simulink model "kuka_sim"  (R2018b)
settings: Solver=VariableStepAuto  StartTime=0.0  StopTime=20  RelTol=1e-3
model workspace (MAT data in the model file):
  MCOS : class17 (value not decoded)
  MCOS : class17 (value not decoded)
  MCOS : class17 (value not decoded)
  MCOS : class17 (value not decoded)
  MCOS : class17 (value not decoded)
  MCOS : class17 (value not decoded)
  MCOS : class17 (value not decoded)
  I_C_1 = [0.00455  0  0; 0  0.00454  1e-05; 0  -1e-05  0.00029]
  I_C_2 = [0.00032  0  0; 0  0.0001  0; 0  0  0.00042]
  I_C_3 = [0.00223  -5e-05  7e-05; 5e-05  0.00219  7e-05; -7e-05  -7e-05  0.00073]
  I_C_4 = [0.03844  0.00088  -0.00112; -0.00088  0.01144  -0.00111; 0.00112  0.00111  0.04988]
  I_C_5 = [0.00277  -1e-05  1e-05; 1e-05  0.00284  0; -1e-05  0  0.00012]
  I_C_6 = [0.0005  -5e-05  -3e-05; 5e-05  0.00281  -4e-05; 3e-05  4e-05  0.00232]
  I_C_7 = [0.00795  0.00022  -0.00029; -0.00022  0.01089  -0.00029; 0.00029  0.00029  0.00294]
  MCOS : class17 (value not decoded)
  MCOS : class17 (value not decoded)
  MCOS : class17 (value not decoded)
  MCOS : class17 (value not decoded)
  MCOS : class17 (value not decoded)
  MCOS : class17 (value not decoded)
  MCOS : class17 (value not decoded)
  Pc_1 = [-0.00351; 0.0016; -0.03139]
  Pc_2 = [-0.00767; 0.16669; -0.00355]
  Pc_3 = [-0.00225; -0.03492; -0.02652]
  Pc_4 = [0.0002; -0.05268; 0.03818]
  Pc_5 = [5e-05; -0.00237; -0.21134]
  Pc_6 = [0.00049; 0.02019; -0.0275]
  Pc_7 = [-0.03466; -0.02324; 0.07138]
  MCOS : class17 (value not decoded)
  MCOS : class17 (value not decoded)
  MCOS : class17 (value not decoded)
  MCOS : class17 (value not decoded)
  MCOS : class17 (value not decoded)
  MCOS : class17 (value not decoded)
  MCOS : class17 (value not decoded)
  MCOS : class17 (value not decoded)
  MCOS : class17 (value not decoded)
  MCOS : class17 (value not decoded)
  MCOS : class17 (value not decoded)
  MCOS : class17 (value not decoded)
  MCOS : class17 (value not decoded)
  MCOS : class17 (value not decoded)
  MCOS : class17 (value not decoded)
  T_8_7 = [1 0 0 0 0 1 0 0 0 0 1 0 ... (16 elements, 4x4)]
  V_0 = [0; 0; 0]
  MCOS : class17 (value not decoded)
  MCOS : class17 (value not decoded)
  MCOS : class17 (value not decoded)
  MCOS : class17 (value not decoded)
  MCOS : class17 (value not decoded)
  MCOS : class17 (value not decoded)
  MCOS : class17 (value not decoded)
  MCOS : class17 (value not decoded)
  MCOS : class17 (value not decoded)
  MCOS : class17 (value not decoded)
  MCOS : class17 (value not decoded)
  MCOS : class17 (value not decoded)
  MCOS : class17 (value not decoded)
  MCOS : class17 (value not decoded)
  MCOS : class17 (value not decoded)
  MCOS : class17 (value not decoded)
  MCOS : class17 (value not decoded)
  MCOS : class17 (value not decoded)
  MCOS : class17 (value not decoded)
  MCOS : class17 (value not decoded)
  MCOS : class17 (value not decoded)
  MCOS : class17 (value not decoded)
  Var1 = 0
  W_0 = [0; 0; 0]
  W_0_dot = [0; 0; 0]
  MCOS : class17 (value not decoded)
  MCOS : class17 (value not decoded)
  MCOS : class17 (value not decoded)
  MCOS : class17 (value not decoded)
  MCOS : class17 (value not decoded)
  MCOS : class17 (value not decoded)
  MCOS : class17 (value not decoded)
  MCOS : class17 (value not decoded)
  MCOS : class17 (value not decoded)
  MCOS : class17 (value not decoded)
  MCOS : class17 (value not decoded)
  MCOS : class17 (value not decoded)
  MCOS : class17 (value not decoded)
  MCOS : class17 (value not decoded)
  a_0 = 0
  a_1 = 0
  a_2 = 0
  a_3 = 0
  a_4 = 0
  a_5 = 0
  a_6 = 0
  a_7 = 0
  alpha_0 = 0
  alpha_1 = 90
  alpha_2 = -90
  alpha_3 = -90
  alpha_4 = 90
  alpha_5 = 90
  alpha_6 = -90
  alpha_7 = 0
  d_1 = 0
  d_2 = 0
  d_3 = 0.4
  d_4 = 0
  d_5 = 0.39
  d_6 = 0
  d_7 = 0
  d_8 = 0
  MCOS : class17 (value not decoded)
  MCOS : class17 (value not decoded)
  MCOS : class17 (value not decoded)
  MCOS : class17 (value not decoded)
  MCOS : class17 (value not decoded)
  MCOS : class17 (value not decoded)
  MCOS : class17 (value not decoded)
  f_end = [0; 0; 0]
  MCOS : class17 (value not decoded)
  m1 = 3.94781
  m2 = 4.50275
  m3 = 2.4552
  m4 = 2.61155
  m5 = 3.41
  m6 = 3.38795
  m7 = 0.35432
  MCOS : class17 (value not decoded)
  MCOS : class17 (value not decoded)
  MCOS : class17 (value not decoded)
  MCOS : class17 (value not decoded)
  MCOS : class17 (value not decoded)
  MCOS : class17 (value not decoded)
  MCOS : class17 (value not decoded)
  n_end = [0; 0; 0]
  pi = 180
  MCOS : class17 (value not decoded)
  MCOS : class17 (value not decoded)
  MCOS : class17 (value not decoded)
  MCOS : class17 (value not decoded)
  MCOS : class17 (value not decoded)
  MCOS : class17 (value not decoded)
  MCOS : class17 (value not decoded)
  MCOS : class17 (value not decoded)
  MCOS : class17 (value not decoded)
  MCOS : class17 (value not decoded)
  MCOS : class17 (value not decoded)
  MCOS : class17 (value not decoded)
  MCOS : class17 (value not decoded)
  MCOS : class17 (value not decoded)
  MCOS : class17 (value not decoded)
  MCOS : class17 (value not decoded)
  MCOS : class17 (value not decoded)
  MCOS : class17 (value not decoded)
  MCOS : class17 (value not decoded)
  MCOS : class17 (value not decoded)
  MCOS : class17 (value not decoded)
  MCOS : class17 (value not decoded)
  MCOS : class17 (value not decoded)
  MCOS : class17 (value not decoded)
  MCOS : class17 (value not decoded)
  MCOS : class17 (value not decoded)
  MCOS : class17 (value not decoded)
  MCOS : class17 (value not decoded)
  MCOS : class17 (value not decoded)
  MCOS : class17 (value not decoded)
  MCOS : class17 (value not decoded)
  MCOS : class17 (value not decoded)
  MCOS : class17 (value not decoded)
  MCOS : class17 (value not decoded)
  MCOS : class17 (value not decoded)
  theta_8 = 0
(part 2 of 2)

== matlab function kuka_sim/MATLAB Function2 ==
  data: q input; torque output; q_dot input; q_des input; q_des_dot input; q_des_ddot input
function torque = fcn(q,q_dot,q_des,q_des_dot,q_des_ddot)

q_1 = q(1);
q_2 = q(2);
q_3 = q(3);
q_4 = q(4);

q_1_dot = q_dot(1);
q_2_dot = q_dot(2);
q_3_dot = q_dot(3);
q_4_dot = q_dot(4);

% q_1_ddot = q_ddot(1);
% q_2_ddot = q_ddot(2);
% q_3_ddot = q_ddot(3);
% q_4_ddot = q_ddot(4);

m11=cos(q_2)*(0.00415795377963*cos(q_2) + 0.005756821258825*sin(q_2) + 0.001993178216*cos(q_3)*sin(q_2) - 0.03195052591232*sin(q_2)*sin(q_3) + 1.0*cos(q_4)*(0.01524699328022*cos(q_2)*cos(q_4) - 0.000208924*cos(q_3)*sin(q_2) - 0.0008524847092*cos(q_2)*sin(q_4) + 0.00414266901372*sin(q_2)*sin(q_3) + 0.0008524847092*cos(q_3)*cos(q_4)*sin(q_2) + 0.01524699328022*cos(q_3)*sin(q_2)*sin(q_4) + 0.0398835916*cos(q_4)*sin(q_2)*sin(q_3)) + sin(q_4)*(0.0009075152908*cos(q_2)*cos(q_4) - 0.0550305816*cos(q_3)*sin(q_2) + 0.04949441641494*cos(q_2)*sin(q_4) - 0.0011399417958*sin(q_2)*sin(q_3) + 0.0398835916*sin(q_2)*sin(q_3)*sin(q_4) - 0.04949441641494*cos(q_3)*cos(q_4)*sin(q_2) + 0.0009075152908*cos(q_3)*sin(q_2)*sin(q_4))) + 1.0*sin(q_2)*(0.005756821258825*cos(q_2) + 0.12548815863615*sin(q_2) - 1.0*cos(q_3)*(0.000076501784*cos(q_2) + 0.01909410731264*cos(q_3)*sin(q_2) - 0.000242905064*sin(q_2)*sin(q_3) + 1.0*cos(q_4)*(0.0009075152908*cos(q_2)*cos(q_4) - 0.0550305816*cos(q_3)*sin(q_2) + 0.04949441641494*cos(q_2)*sin(q_4) - 0.0011399417958*sin(q_2)*sin(q_3) + 0.0398835916*sin(q_2)*sin(q_3)*sin(q_4) - 0.04949441641494*cos(q_3)*cos(q_4)*sin(q_2) + 0.0009075152908*cos(q_3)*sin(q_2)*sin(q_4)) - 1.0*sin(q_4)*(0.01524699328022*cos(q_2)*cos(q_4) - 0.000208924*cos(q_3)*sin(q_2) - 0.0008524847092*cos(q_2)*sin(q_4) + 0.00414266901372*sin(q_2)*sin(q_3) + 0.0008524847092*cos(q_3)*cos(q_4)*sin(q_2) + 0.01524699328022*cos(q_3)*sin(q_2)*sin(q_4) + 0.0398835916*cos(q_4)*sin(q_2)*sin(q_3))) + 1.0*sin(q_3)*(0.00220370768768*cos(q_2) + 0.00636266901372*cos(q_2)*cos(q_4) + 0.000142905064*cos(q_3)*sin(q_2) + 0.0011000582042*cos(q_2)*sin(q_4) + 0.0350120676028*sin(q_2)*sin(q_3) - 0.000208924*sin(q_2)*sin(q_3)*sin(q_4) - 0.0011000582042*cos(q_3)*cos(q_4)*sin(q_2) + 0.00636266901372*cos(q_3)*sin(q_2)*sin(q_4) + 0.0550305816*cos(q_4)*sin(q_2)*sin(q_3)) + 0.4*sin(q_3)*(cos(q_4)*(0.099708979*cos(q_2)*cos(q_4) + 0.137576454*sin(q_2)*sin(q_3) + 0.099708979*cos(q_3)*sin(q_2)*sin(q_4) + 1.04462*cos(q_4)*sin(q_2)*sin(q_3)) - 0.085735584*cos(q_2) + 0.916968096*sin(q_2)*sin(q_3) + 1.0*sin(q_4)*(0.099708979*cos(q_2)*sin(q_4) - 0.00052231*sin(q_2)*sin(q_3) + 1.04462*sin(q_2)*sin(q_3)*sin(q_4) - 0.099708979*cos(q_3)*cos(q_4)*sin(q_2))) + 0.4*cos(q_3)*(0.0055242*cos(q_2) - 0.00052231*cos(q_2)*cos(q_4) + 1.961588096*cos(q_3)*sin(q_2) - 0.137576454*cos(q_2)*sin(q_4) + 0.137576454*cos(q_3)*cos(q_4)*sin(q_2) - 0.00052231*cos(q_3)*sin(q_2)*sin(q_4))) + 0.00034874380758100000061534551321074;
m12=1.0*sin(q_2)*(1.0*cos(q_3)*(0.000242905064*cos(q_3) + 0.01909410731264*sin(q_3) - 1.0*cos(q_4)*(0.0550305816*sin(q_3) - 0.0011399417958*cos(q_3) + 0.0398835916*cos(q_3)*sin(q_4) + 0.04949441641494*cos(q_4)*sin(q_3) - 0.0009075152908*sin(q_3)*sin(q_4)) + 1.0*sin(q_4)*(0.00414266901372*cos(q_3) + 0.000208924*sin(q_3) + 0.0398835916*cos(q_3)*cos(q_4) - 0.0008524847092*cos(q_4)*sin(q_3) - 0.01524699328022*sin(q_3)*sin(q_4))) - 0.4*cos(q_3)*(1.961588096*sin(q_3) + 0.137576454*cos(q_4)*sin(q_3) - 0.00052231*sin(q_3)*sin(q_4)) + 0.4*sin(q_3)*(0.916968096*cos(q_3) + cos(q_4)*(0.137576454*cos(q_3) + 1.04462*cos(q_3)*cos(q_4) - 0.099708979*sin(q_3)*sin(q_4)) + 1.0*sin(q_4)*(1.04462*cos(q_3)*sin(q_4) - 0.00052231*cos(q_3) + 0.099708979*cos(q_4)*sin(q_3))) + 1.0*sin(q_3)*(0.0350120676028*cos(q_3) - 0.000142905064*sin(q_3) + 0.0550305816*cos(q_3)*cos(q_4) - 0.000208924*cos(q_3)*sin(q_4) + 0.0011000582042*cos(q_4)*sin(q_3) - 0.00636266901372*sin(q_3)*sin(q_4)) - 0.000122603128375) + cos(q_2)*(1.0*cos(q_4)*(0.00414266901372*cos(q_3) + 0.000208924*sin(q_3) + 0.0398835916*cos(q_3)*cos(q_4) - 0.0008524847092*cos(q_4)*sin(q_3) - 0.01524699328022*sin(q_3)*sin(q_4)) - 0.001993178216*sin(q_3) - 0.03195052591232*cos(q_3) + sin(q_4)*(0.0550305816*sin(q_3) - 0.0011399417958*cos(q_3) + 0.0398835916*cos(q_3)*sin(q_4) + 0.04949441641494*cos(q_4)*sin(q_3) - 0.0009075152908*sin(q_3)*sin(q_4)) + 0.002664500061125);
m13=cos(q_2)*(sin(q_4)*(0.0009075152908*cos(q_4) + 0.04949441641494*sin(q_4)) + 1.0*cos(q_4)*(0.01524699328022*cos(q_4) - 0.0008524847092*sin(q_4)) + 0.00373631604328) + 1.0*sin(q_2)*(1.0*sin(q_3)*(0.00636266901372*cos(q_4) + 0.0011000582042*sin(q_4) + 0.00220370768768) - 1.0*cos(q_3)*(1.0*cos(q_4)*(0.0009075152908*cos(q_4) + 0.04949441641494*sin(q_4)) - 1.0*sin(q_4)*(0.01524699328022*cos(q_4) - 0.0008524847092*sin(q_4)) + 0.000076501784) - 0.4*cos(q_3)*(0.00052231*cos(q_4) + 0.137576454*sin(q_4) - 0.0055242) + 0.4*sin(q_3)*(0.099708979*cos(q_4)^2 + 0.099708979*sin(q_4)^2 - 0.085735584));
m14=- 1.0*sin(q_2)*(0.05712763205872*sin(q_3) + 1.0*cos(q_3)*(0.0011399417958*cos(q_4) + 0.00414266901372*sin(q_4)) + 0.4*sin(q_3)*(0.137576454*cos(q_4) - 0.00052231*sin(q_4))) - cos(q_2)*(0.00414266901372*cos(q_4) - 0.0011399417958*sin(q_4));
m21=0.002664500061125*cos(q_2) - 0.000122603128375*sin(q_2) + sin(q_3)*(0.000076501784*cos(q_2) + 0.01909410731264*cos(q_3)*sin(q_2) - 0.000242905064*sin(q_2)*sin(q_3) + 1.0*cos(q_4)*(0.0009075152908*cos(q_2)*cos(q_4) - 0.0550305816*cos(q_3)*sin(q_2) + 0.04949441641494*cos(q_2)*sin(q_4) - 0.0011399417958*sin(q_2)*sin(q_3) + 0.0398835916*sin(q_2)*sin(q_3)*sin(q_4) - 0.04949441641494*cos(q_3)*cos(q_4)*sin(q_2) + 0.0009075152908*cos(q_3)*sin(q_2)*sin(q_4)) - 1.0*sin(q_4)*(0.01524699328022*cos(q_2)*cos(q_4) - 0.000208924*cos(q_3)*sin(q_2) - 0.0008524847092*cos(q_2)*sin(q_4) + 0.00414266901372*sin(q_2)*sin(q_3) + 0.0008524847092*cos(q_3)*cos(q_4)*sin(q_2) + 0.01524699328022*cos(q_3)*sin(q_2)*sin(q_4) + 0.0398835916*cos(q_4)*sin(q_2)*sin(q_3))) + 1.0*cos(q_3)*(0.00220370768768*cos(q_2) + 0.00636266901372*cos(q_2)*cos(q_4) + 0.000142905064*cos(q_3)*sin(q_2) + 0.0011000582042*cos(q_2)*sin(q_4) + 0.0350120676028*sin(q_2)*sin(q_3) - 0.000208924*sin(q_2)*sin(q_3)*sin(q_4) - 0.0011000582042*cos(q_3)*cos(q_4)*sin(q_2) + 0.00636266901372*cos(q_3)*sin(q_2)*sin(q_4) + 0.0550305816*cos(q_4)*sin(q_2)*sin(q_3)) + 0.4*cos(q_3)*(cos(q_4)*(0.099708979*cos(q_2)*cos(q_4) + 0.137576454*sin(q_2)*sin(q_3) + 0.099708979*cos(q_3)*sin(q_2)*sin(q_4) + 1.04462*cos(q_4)*sin(q_2)*sin(q_3)) - 0.085735584*cos(q_2) + 0.916968096*sin(q_2)*sin(q_3) + 1.0*sin(q_4)*(0.099708979*cos(q_2)*sin(q_4) - 0.00052231*sin(q_2)*sin(q_3) + 1.04462*sin(q_2)*sin(q_3)*sin(q_4) - 0.099708979*cos(q_3)*cos(q_4)*sin(q_2))) - 0.4*sin(q_3)*(0.0055242*cos(q_2) - 0.00052231*cos(q_2)*cos(q_4) + 1.961588096*cos(q_3)*sin(q_2) - 0.137576454*cos(q_2)*sin(q_4) + 0.137576454*cos(q_3)*cos(q_4)*sin(q_2) - 0.00052231*cos(q_3)*sin(q_2)*sin(q_4));
m22=0.4*sin(q_3)*(1.961588096*sin(q_3) + 0.137576454*cos(q_4)*sin(q_3) - 0.00052231*sin(q_3)*sin(q_4)) - sin(q_3)*(0.000242905064*cos(q_3) + 0.01909410731264*sin(q_3) - 1.0*cos(q_4)*(0.0550305816*sin(q_3) - 0.0011399417958*cos(q_3) + 0.0398835916*cos(q_3)*sin(q_4) + 0.04949441641494*cos(q_4)*sin(q_3) - 0.0009075152908*sin(q_3)*sin(q_4)) + 1.0*sin(q_4)*(0.00414266901372*cos(q_3) + 0.000208924*sin(q_3) + 0.0398835916*cos(q_3)*cos(q_4) - 0.0008524847092*cos(q_4)*sin(q_3) - 0.01524699328022*sin(q_3)*sin(q_4))) + 0.4*cos(q_3)*(0.916968096*cos(q_3) + cos(q_4)*(0.137576454*cos(q_3) + 1.04462*cos(q_3)*cos(q_4) - 0.099708979*sin(q_3)*sin(q_4)) + 1.0*sin(q_4)*(1.04462*cos(q_3)*sin(q_4) - 0.00052231*cos(q_3) + 0.099708979*cos(q_4)*sin(q_3))) + 1.0*cos(q_3)*(0.0350120676028*cos(q_3) - 0.000142905064*sin(q_3) + 0.0550305816*cos(q_3)*cos(q_4) - 0.000208924*cos(q_3)*sin(q_4) + 0.0011000582042*cos(q_4)*sin(q_3) - 0.00636266901372*sin(q_3)*sin(q_4)) + 0.12579630455875;
m23=0.4*sin(q_3)*(0.00052231*cos(q_4) + 0.137576454*sin(q_4) - 0.0055242) + 1.0*cos(q_3)*(0.00636266901372*cos(q_4) + 0.0011000582042*sin(q_4) + 0.00220370768768) + sin(q_3)*(1.0*cos(q_4)*(0.0009075152908*cos(q_4) + 0.04949441641494*sin(q_4)) - 1.0*sin(q_4)*(0.01524699328022*cos(q_4) - 0.0008524847092*sin(q_4)) + 0.000076501784) + 0.4*cos(q_3)*(0.099708979*cos(q_4)^2 + 0.099708979*sin(q_4)^2 - 0.085735584);
m24=sin(q_3)*(0.0011399417958*cos(q_4) + 0.00414266901372*sin(q_4)) - 0.4*cos(q_3)*(0.137576454*cos(q_4) - 0.00052231*sin(q_4)) - 0.05712763205872*cos(q_3);
m31=0.00373631604328*cos(q_2) + 0.001993178216*cos(q_3)*sin(q_2) - 0.03195052591232*sin(q_2)*sin(q_3) + 1.0*cos(q_4)*(0.01524699328022*cos(q_2)*cos(q_4) - 0.000208924*cos(q_3)*sin(q_2) - 0.0008524847092*cos(q_2)*sin(q_4) + 0.00414266901372*sin(q_2)*sin(q_3) + 0.0008524847092*cos(q_3)*cos(q_4)*sin(q_2) + 0.01524699328022*cos(q_3)*sin(q_2)*sin(q_4) + 0.0398835916*cos(q_4)*sin(q_2)*sin(q_3)) + sin(q_4)*(0.0009075152908*cos(q_2)*cos(q_4) - 0.0550305816*cos(q_3)*sin(q_2) + 0.04949441641494*cos(q_2)*sin(q_4) - 0.0011399417958*sin(q_2)*sin(q_3) + 0.0398835916*sin(q_2)*sin(q_3)*sin(q_4) - 0.04949441641494*cos(q_3)*cos(q_4)*sin(q_2) + 0.0009075152908*cos(q_3)*sin(q_2)*sin(q_4));
m32=1.0*cos(q_4)*(0.00414266901372*cos(q_3) + 0.000208924*sin(q_3) + 0.0398835916*cos(q_3)*cos(q_4) - 0.0008524847092*cos(q_4)*sin(q_3) - 0.01524699328022*sin(q_3)*sin(q_4)) - 0.001993178216*sin(q_3) - 0.03195052591232*cos(q_3) + sin(q_4)*(0.0550305816*sin(q_3) - 0.0011399417958*cos(q_3) + 0.0398835916*cos(q_3)*sin(q_4) + 0.04949441641494*cos(q_4)*sin(q_3) - 0.0009075152908*sin(q_3)*sin(q_4));
m33=sin(q_4)*(0.0009075152908*cos(q_4) + 0.04949441641494*sin(q_4)) + 1.0*cos(q_4)*(0.01524699328022*cos(q_4) - 0.0008524847092*sin(q_4)) + 0.00373631604328;
m34=0.0011399417958*sin(q_4) - 0.00414266901372*cos(q_4);
m41=0.000208924*sin(q_2)*sin(q_3)*sin(q_4) - 0.0011000582042*cos(q_2)*sin(q_4) - 0.05712763205872*sin(q_2)*sin(q_3) - 0.00636266901372*cos(q_2)*cos(q_4) + 0.0011000582042*cos(q_3)*cos(q_4)*sin(q_2) - 0.00636266901372*cos(q_3)*sin(q_2)*sin(q_4) - 0.0550305816*cos(q_4)*sin(q_2)*sin(q_3);
m42=0.000208924*cos(q_3)*sin(q_4) - 0.0550305816*cos(q_3)*cos(q_4) - 0.05712763205872*cos(q_3) - 0.0011000582042*cos(q_4)*sin(q_3) + 0.00636266901372*sin(q_3)*sin(q_4);
m43=- 0.00636266901372*cos(q_4) - 0.0011000582042*sin(q_4);
m44=0.05712763205872;

M=[m11 m12 m13 m14;m21 m22 m23 m24;m31 m32 m33 m34;m41 m42 m43 m44];

c11=0;
c12=- cos(q_2)*(0.005756821258825*q_1*sin(q_2)^2 + 0.0055242*cos(q_3)*(0.4*q_1*sin(q_2)^2 - 0.4*q_2*cos(q_2)) - 0.085735584*sin(q_3)*(0.4*q_1*sin(q_2)^2 - 0.4*q_2*cos(q_2)) + 1.0*cos(q_4)*(0.01524699328022*cos(q_4)*(1.0*q_2*sin(q_2) + 1.0*q_1*cos(q_2)*sin(q_2)) - 0.00052231*cos(q_3)*(0.4*q_1*sin(q_2)^2 - 0.4*q_2*cos(q_2)) - 0.0008524847092*sin(q_4)*(1.0*q_2*sin(q_2) + 1.0*q_1*cos(q_2)*sin(q_2)) + 0.00414266901372*sin(q_3)*(1.0*q_1*sin(q_2)^2 - 1.0*q_2*cos(q_2)) + 0.0008524847092*cos(q_3)*cos(q_4)*(1.0*q_1*sin(q_2)^2 - 1.0*q_2*cos(q_2)) + 0.01524699328022*cos(q_3)*sin(q_4)*(1.0*q_1*sin(q_2)^2 - 1.0*q_2*cos(q_2)) + 0.099708979*cos(q_4)*sin(q_3)*(0.4*q_1*sin(q_2)^2 - 0.4*q_2*cos(q_2))) + sin(q_4)*(0.0009075152908*cos(q_4)*(1.0*q_2*sin(q_2) + 1.0*q_1*cos(q_2)*sin(q_2)) - 0.137576454*cos(q_3)*(0.4*q_1*sin(q_2)^2 - 0.4*q_2*cos(q_2)) + 0.04949441641494*sin(q_4)*(1.0*q_2*sin(q_2) + 1.0*q_1*cos(q_2)*sin(q_2)) - 0.0011399417958*sin(q_3)*(1.0*q_1*sin(q_2)^2 - 1.0*q_2*cos(q_2)) + 0.099708979*sin(q_3)*sin(q_4)*(0.4*q_1*sin(q_2)^2 - 0.4*q_2*cos(q_2)) - 0.04949441641494*cos(q_3)*cos(q_4)*(1.0*q_1*sin(q_2)^2 - 1.0*q_2*cos(q_2)) + 0.0009075152908*cos(q_3)*sin(q_4)*(1.0*q_1*sin(q_2)^2 - 1.0*q_2*cos(q_2))) - 0.005756821258825*q_2*cos(q_2) + 0.00415795377963*q_2*sin(q_2) - 0.000216501784*cos(q_3)*(1.0*q_1*sin(q_2)^2 - 1.0*q_2*cos(q_2)) + 0.00234370768768*sin(q_3)*(1.0*q_1*sin(q_2)^2 - 1.0*q_2*cos(q_2)) + 0.00415795377963*q_1*cos(q_2)*sin(q_2)) - 1.0*sin(q_2)*(0.12548815863615*q_1*sin(q_2)^2 + 0.4*cos(q_3)*(5.06675*cos(q_3)*(0.4*q_1*sin(q_2)^2 - 0.4*q_2*cos(q_2)) - 0.00052231*cos(q_4)*(1.0*q_2*sin(q_2) + 1.0*q_1*cos(q_2)*sin(q_2)) - 0.137576454*sin(q_4)*(1.0*q_2*sin(q_2) + 1.0*q_1*cos(q_2)*sin(q_2)) + 0.0055242*q_2*sin(q_2) - 0.065111904*cos(q_3)*(1.0*q_1*sin(q_2)^2 - 1.0*q_2*cos(q_2)) + 0.0055242*q_1*cos(q_2)*sin(q_2) + 0.137576454*cos(q_3)*cos(q_4)*(1.0*q_1*sin(q_2)^2 - 1.0*q_2*cos(q_2)) - 0.00052231*cos(q_3)*sin(q_4)*(1.0*q_1*sin(q_2)^2 - 1.0*q_2*cos(q_2))) + 0.4*sin(q_3)*(2.4552*sin(q_3)*(0.4*q_1*sin(q_2)^2 - 0.4*q_2*cos(q_2)) - 0.085735584*q_2*sin(q_2) - 0.065111904*sin(q_3)*(1.0*q_1*sin(q_2)^2 - 1.0*q_2*cos(q_2)) + cos(q_4)*(0.099708979*cos(q_4)*(1.0*q_2*sin(q_2) + 1.0*q_1*cos(q_2)*sin(q_2)) + 0.137576454*sin(q_3)*(1.0*q_1*sin(q_2)^2 - 1.0*q_2*cos(q_2)) + 0.099708979*cos(q_3)*sin(q_4)*(1.0*q_1*sin(q_2)^2 - 1.0*q_2*cos(q_2)) + 2.61155*cos(q_4)*sin(q_3)*(0.4*q_1*sin(q_2)^2 - 0.4*q_2*cos(q_2))) + 1.0*sin(q_4)*(0.099708979*sin(q_4)*(1.0*q_2*sin(q_2) + 1.0*q_1*cos(q_2)*sin(q_2)) - 0.00052231*sin(q_3)*(1.0*q_1*sin(q_2)^2 - 1.0*q_2*cos(q_2)) + 2.61155*sin(q_3)*sin(q_4)*(0.4*q_1*sin(q_2)^2 - 0.4*q_2*cos(q_2)) - 0.099708979*cos(q_3)*cos(q_4)*(1.0*q_1*sin(q_2)^2 - 1.0*q_2*cos(q_2))) - 0.085735584*q_1*cos(q_2)*sin(q_2)) + 1.0*sin(q_3)*(0.00636266901372*cos(q_4)*(1.0*q_2*sin(q_2) + 1.0*q_1*cos(q_2)*sin(q_2)) - 0.065111904*sin(q_3)*(0.4*q_1*sin(q_2)^2 - 0.4*q_2*cos(q_2)) + 0.0011000582042*sin(q_4)*(1.0*q_2*sin(q_2) + 1.0*q_1*cos(q_2)*sin(q_2)) + 0.00220370768768*q_2*sin(q_2) + 0.000142905064*cos(q_3)*(1.0*q_1*sin(q_2)^2 - 1.0*q_2*cos(q_2)) + 0.0610568292028*sin(q_3)*(1.0*q_1*sin(q_2)^2 - 1.0*q_2*cos(q_2)) - 0.00052231*sin(q_3)*sin(q_4)*(0.4*q_1*sin(q_2)^2 - 0.4*q_2*cos(q_2)) + 0.00220370768768*q_1*cos(q_2)*sin(q_2) - 0.0011000582042*cos(q_3)*cos(q_4)*(1.0*q_1*sin(q_2)^2 - 1.0*q_2*cos(q_2)) + 0.00636266901372*cos(q_3)*sin(q_4)*(1.0*q_1*sin(q_2)^2 - 1.0*q_2*cos(q_2)) + 0.137576454*cos(q_4)*sin(q_3)*(0.4*q_1*sin(q_2)^2 - 0.4*q_2*cos(q_2))) - 0.12548815863615*q_2*cos(q_2) + 0.005756821258825*q_2*sin(q_2) - 1.0*cos(q_3)*(0.065111904*cos(q_3)*(0.4*q_1*sin(q_2)^2 - 0.4*q_2*cos(q_2)) + 1.0*cos(q_4)*(0.0009075152908*cos(q_4)*(1.0*q_2*sin(q_2) + 1.0*q_1*cos(q_2)*sin(q_2)) - 0.137576454*cos(q_3)*(0.4*q_1*sin(q_2)^2 - 0.4*q_2*cos(q_2)) + 0.04949441641494*sin(q_4)*(1.0*q_2*sin(q_2) + 1.0*q_1*cos(q_2)*sin(q_2)) - 0.0011399417958*sin(q_3)*(1.0*q_1*sin(q_2)^2 - 1.0*q_2*cos(q_2)) + 0.099708979*sin(q_3)*sin(q_4)*(0.4*q_1*sin(q_2)^2 - 0.4*q_2*cos(q_2)) - 0.04949441641494*cos(q_3)*cos(q_4)*(1.0*q_1*sin(q_2)^2 - 1.0*q_2*cos(q_2)) + 0.0009075152908*cos(q_3)*sin(q_4)*(1.0*q_1*sin(q_2)^2 - 1.0*q_2*cos(q_2))) - 1.0*sin(q_4)*(0.01524699328022*cos(q_4)*(1.0*q_2*sin(q_2) + 1.0*q_1*cos(q_2)*sin(q_2)) - 0.00052231*cos(q_3)*(0.4*q_1*sin(q_2)^2 - 0.4*q_2*cos(q_2)) - 0.0008524847092*sin(q_4)*(1.0*q_2*sin(q_2) + 1.0*q_1*cos(q_2)*sin(q_2)) + 0.00414266901372*sin(q_3)*(1.0*q_1*sin(q_2)^2 - 1.0*q_2*cos(q_2)) + 0.0008524847092*cos(q_3)*cos(q_4)*(1.0*q_1*sin(q_2)^2 - 1.0*q_2*cos(q_2)) + 0.01524699328022*cos(q_3)*sin(q_4)*(1.0*q_1*sin(q_2)^2 - 1.0*q_2*cos(q_2)) + 0.099708979*cos(q_4)*sin(q_3)*(0.4*q_1*sin(q_2)^2 - 0.4*q_2*cos(q_2))) + 0.000076501784*q_2*sin(q_2) - 0.00695065428736*cos(q_3)*(1.0*q_1*sin(q_2)^2 - 1.0*q_2*cos(q_2)) - 0.000242905064*sin(q_3)*(1.0*q_1*sin(q_2)^2 - 1.0*q_2*cos(q_2)) + 0.000076501784*q_1*cos(q_2)*sin(q_2)) + 0.005756821258825*q_1*cos(q_2)*sin(q_2));
c13=- 1.0*sin(q_2)*(0.4*cos(q_3)*(0.065111904*sin(q_3)*(q_2*sin(q_3) - 1.0*q_1*cos(q_3)*sin(q_2)) - 0.065111904*cos(q_3)*(q_3 + q_1*cos(q_2)) - 0.137576454*cos(q_4)*(1.0*sin(q_3)*(q_2*sin(q_3) - 1.0*q_1*cos(q_3)*sin(q_2)) - 1.0*cos(q_3)*(q_3 + q_1*cos(q_2))) + 0.00052231*sin(q_4)*(1.0*sin(q_3)*(q_2*sin(q_3) - 1.0*q_1*cos(q_3)*sin(q_2)) - 1.0*cos(q_3)*(q_3 + q_1*cos(q_2)))) + 1.0*sin(q_3)*(0.0610568292028*cos(q_3)*(q_2*sin(q_3) - 1.0*q_1*cos(q_3)*sin(q_2)) - 0.000142905064*sin(q_3)*(q_2*sin(q_3) - 1.0*q_1*cos(q_3)*sin(q_2)) + 0.000142905064*cos(q_3)*(q_3 + q_1*cos(q_2)) + 0.0610568292028*sin(q_3)*(q_3 + q_1*cos(q_2)) + 0.0011000582042*cos(q_4)*(1.0*sin(q_3)*(q_2*sin(q_3) - 1.0*q_1*cos(q_3)*sin(q_2)) - 1.0*cos(q_3)*(q_3 + q_1*cos(q_2))) - 0.00636266901372*sin(q_4)*(1.0*sin(q_3)*(q_2*sin(q_3) - 1.0*q_1*cos(q_3)*sin(q_2)) - 1.0*cos(q_3)*(q_3 + q_1*cos(q_2)))) - 0.4*sin(q_3)*(0.065111904*cos(q_3)*(q_2*sin(q_3) - 1.0*q_1*cos(q_3)*sin(q_2)) + 1.0*sin(q_4)*(0.00052231*cos(q_3)*(q_2*sin(q_3) - 1.0*q_1*cos(q_3)*sin(q_2)) + 0.00052231*sin(q_3)*(q_3 + q_1*cos(q_2)) - 0.099708979*cos(q_4)*(1.0*sin(q_3)*(q_2*sin(q_3) - 1.0*q_1*cos(q_3)*sin(q_2)) - 1.0*cos(q_3)*(q_3 + q_1*cos(q_2)))) - cos(q_4)*(0.137576454*cos(q_3)*(q_2*sin(q_3) - 1.0*q_1*cos(q_3)*sin(q_2)) + 0.137576454*sin(q_3)*(q_3 + q_1*cos(q_2)) - 0.099708979*sin(q_4)*(1.0*sin(q_3)*(q_2*sin(q_3) - 1.0*q_1*cos(q_3)*sin(q_2)) - 1.0*cos(q_3)*(q_3 + q_1*cos(q_2)))) + 0.065111904*sin(q_3)*(q_3 + q_1*cos(q_2))) + 1.0*cos(q_3)*(0.000242905064*cos(q_3)*(q_2*sin(q_3) - 1.0*q_1*cos(q_3)*sin(q_2)) - 0.00695065428736*sin(q_3)*(q_2*sin(q_3) - 1.0*q_1*cos(q_3)*sin(q_2)) + 1.0*cos(q_4)*(0.0011399417958*cos(q_3)*(q_2*sin(q_3) - 1.0*q_1*cos(q_3)*sin(q_2)) + 0.0011399417958*sin(q_3)*(q_3 + q_1*cos(q_2)) - 0.04949441641494*cos(q_4)*(1.0*sin(q_3)*(q_2*sin(q_3) - 1.0*q_1*cos(q_3)*sin(q_2)) - 1.0*cos(q_3)*(q_3 + q_1*cos(q_2))) + 0.0009075152908*sin(q_4)*(1.0*sin(q_3)*(q_2*sin(q_3) - 1.0*q_1*cos(q_3)*sin(q_2)) - 1.0*cos(q_3)*(q_3 + q_1*cos(q_2)))) + 0.00695065428736*cos(q_3)*(q_3 + q_1*cos(q_2)) + 1.0*sin(q_4)*(0.00414266901372*cos(q_3)*(q_2*sin(q_3) - 1.0*q_1*cos(q_3)*sin(q_2)) + 0.00414266901372*sin(q_3)*(q_3 + q_1*cos(q_2)) - 0.0008524847092*cos(q_4)*(1.0*sin(q_3)*(q_2*sin(q_3) - 1.0*q_1*cos(q_3)*sin(q_2)) - 1.0*cos(q_3)*(q_3 + q_1*cos(q_2))) - 0.01524699328022*sin(q_4)*(1.0*sin(q_3)*(q_2*sin(q_3) - 1.0*q_1*cos(q_3)*sin(q_2)) - 1.0*cos(q_3)*(q_3 + q_1*cos(q_2)))) + 0.000242905064*sin(q_3)*(q_3 + q_1*cos(q_2)))) - cos(q_2)*(0.00234370768768*cos(q_3)*(q_2*sin(q_3) - 1.0*q_1*cos(q_3)*sin(q_2)) + 0.000216501784*sin(q_3)*(q_2*sin(q_3) - 1.0*q_1*cos(q_3)*sin(q_2)) + 1.0*cos(q_4)*(0.00414266901372*cos(q_3)*(q_2*sin(q_3) - 1.0*q_1*cos(q_3)*sin(q_2)) + 0.00414266901372*sin(q_3)*(q_3 + q_1*cos(q_2)) - 0.0008524847092*cos(q_4)*(1.0*sin(q_3)*(q_2*sin(q_3) - 1.0*q_1*cos(q_3)*sin(q_2)) - 1.0*cos(q_3)*(q_3 + q_1*cos(q_2))) - 0.01524699328022*sin(q_4)*(1.0*sin(q_3)*(q_2*sin(q_3) - 1.0*q_1*cos(q_3)*sin(q_2)) - 1.0*cos(q_3)*(q_3 + q_1*cos(q_2)))) - 0.000216501784*cos(q_3)*(q_3 + q_1*cos(q_2)) - sin(q_4)*(0.0011399417958*cos(q_3)*(q_2*sin(q_3) - 1.0*q_1*cos(q_3)*sin(q_2)) + 0.0011399417958*sin(q_3)*(q_3 + q_1*cos(q_2)) - 0.04949441641494*cos(q_4)*(1.0*sin(q_3)*(q_2*sin(q_3) - 1.0*q_1*cos(q_3)*sin(q_2)) - 1.0*cos(q_3)*(q_3 + q_1*cos(q_2))) + 0.0009075152908*sin(q_4)*(1.0*sin(q_3)*(q_2*sin(q_3) - 1.0*q_1*cos(q_3)*sin(q_2)) - 1.0*cos(q_3)*(q_3 + q_1*cos(q_2)))) + 0.00234370768768*sin(q_3)*(q_3 + q_1*cos(q_2)));
c14=1.0*sin(q_2)*(1.0*cos(q_3)*(1.0*sin(q_4)*(0.0008524847092*sin(q_4)*(cos(q_4)*(q_2*sin(q_3) - 1.0*q_1*cos(q_3)*sin(q_2)) + sin(q_4)*(q_3 + q_1*cos(q_2))) - 0.01524699328022*cos(q_4)*(cos(q_4)*(q_2*sin(q_3) - 1.0*q_1*cos(q_3)*sin(q_2)) + sin(q_4)*(q_3 + q_1*cos(q_2))) + 0.0008524847092*cos(q_4)*(q_2*cos(q_3) - 1.0*q_4 + q_1*sin(q_2)*sin(q_3)) + 0.01524699328022*sin(q_4)*(q_2*cos(q_3) - 1.0*q_4 + q_1*sin(q_2)*sin(q_3))) + 1.0*cos(q_4)*(0.0009075152908*cos(q_4)*(cos(q_4)*(q_2*sin(q_3) - 1.0*q_1*cos(q_3)*sin(q_2)) + sin(q_4)*(q_3 + q_1*cos(q_2))) + 0.04949441641494*sin(q_4)*(cos(q_4)*(q_2*sin(q_3) - 1.0*q_1*cos(q_3)*sin(q_2)) + sin(q_4)*(q_3 + q_1*cos(q_2))) + 0.04949441641494*cos(q_4)*(q_2*cos(q_3) - 1.0*q_4 + q_1*sin(q_2)*sin(q_3)) - 0.0009075152908*sin(q_4)*(q_2*cos(q_3) - 1.0*q_4 + q_1*sin(q_2)*sin(q_3)))) + 0.4*cos(q_3)*(0.00052231*cos(q_4)*(cos(q_4)*(q_2*sin(q_3) - 1.0*q_1*cos(q_3)*sin(q_2)) + sin(q_4)*(q_3 + q_1*cos(q_2))) + 0.137576454*sin(q_4)*(cos(q_4)*(q_2*sin(q_3) - 1.0*q_1*cos(q_3)*sin(q_2)) + sin(q_4)*(q_3 + q_1*cos(q_2))) + 0.137576454*cos(q_4)*(q_2*cos(q_3) - 1.0*q_4 + q_1*sin(q_2)*sin(q_3)) - 0.00052231*sin(q_4)*(q_2*cos(q_3) - 1.0*q_4 + q_1*sin(q_2)*sin(q_3))) - 0.4*sin(q_3)*(cos(q_4)*(0.099708979*cos(q_4)*(cos(q_4)*(q_2*sin(q_3) - 1.0*q_1*cos(q_3)*sin(q_2)) + sin(q_4)*(q_3 + q_1*cos(q_2))) - 0.099708979*sin(q_4)*(q_2*cos(q_3) - 1.0*q_4 + q_1*sin(q_2)*sin(q_3))) + 1.0*sin(q_4)*(0.099708979*sin(q_4)*(cos(q_4)*(q_2*sin(q_3) - 1.0*q_1*cos(q_3)*sin(q_2)) + sin(q_4)*(q_3 + q_1*cos(q_2))) + 0.099708979*cos(q_4)*(q_2*cos(q_3) - 1.0*q_4 + q_1*sin(q_2)*sin(q_3)))) - 1.0*sin(q_3)*(0.00636266901372*cos(q_4)*(cos(q_4)*(q_2*sin(q_3) - 1.0*q_1*cos(q_3)*sin(q_2)) + sin(q_4)*(q_3 + q_1*cos(q_2))) + 0.0011000582042*sin(q_4)*(cos(q_4)*(q_2*sin(q_3) - 1.0*q_1*cos(q_3)*sin(q_2)) + sin(q_4)*(q_3 + q_1*cos(q_2))) + 0.0011000582042*cos(q_4)*(q_2*cos(q_3) - 1.0*q_4 + q_1*sin(q_2)*sin(q_3)) - 0.00636266901372*sin(q_4)*(q_2*cos(q_3) - 1.0*q_4 + q_1*sin(q_2)*sin(q_3)))) - cos(q_2)*(sin(q_4)*(0.0009075152908*cos(q_4)*(cos(q_4)*(q_2*sin(q_3) - 1.0*q_1*cos(q_3)*sin(q_2)) + sin(q_4)*(q_3 + q_1*cos(q_2))) + 0.04949441641494*sin(q_4)*(cos(q_4)*(q_2*sin(q_3) - 1.0*q_1*cos(q_3)*sin(q_2)) + sin(q_4)*(q_3 + q_1*cos(q_2))) + 0.04949441641494*cos(q_4)*(q_2*cos(q_3) - 1.0*q_4 + q_1*sin(q_2)*sin(q_3)) - 0.0009075152908*sin(q_4)*(q_2*cos(q_3) - 1.0*q_4 + q_1*sin(q_2)*sin(q_3))) - 1.0*cos(q_4)*(0.0008524847092*sin(q_4)*(cos(q_4)*(q_2*sin(q_3) - 1.0*q_1*cos(q_3)*sin(q_2)) + sin(q_4)*(q_3 + q_1*cos(q_2))) - 0.01524699328022*cos(q_4)*(cos(q_4)*(q_2*sin(q_3) - 1.0*q_1*cos(q_3)*sin(q_2)) + sin(q_4)*(q_3 + q_1*cos(q_2))) + 0.0008524847092*cos(q_4)*(q_2*cos(q_3) - 1.0*q_4 + q_1*sin(q_2)*sin(q_3)) + 0.01524699328022*sin(q_4)*(q_2*cos(q_3) - 1.0*q_4 + q_1*sin(q_2)*sin(q_3))));
c21=0;
c22=0.000122603128375*q_1*sin(q_2)^2 + 0.4*sin(q_3)*(5.06675*cos(q_3)*(0.4*q_1*sin(q_2)^2 - 0.4*q_2*cos(q_2)) - 0.00052231*cos(q_4)*(1.0*q_2*sin(q_2) + 1.0*q_1*cos(q_2)*sin(q_2)) - 0.137576454*sin(q_4)*(1.0*q_2*sin(q_2) + 1.0*q_1*cos(q_2)*sin(q_2)) + 0.0055242*q_2*sin(q_2) - 0.065111904*cos(q_3)*(1.0*q_1*sin(q_2)^2 - 1.0*q_2*cos(q_2)) + 0.0055242*q_1*cos(q_2)*sin(q_2) + 0.137576454*cos(q_3)*cos(q_4)*(1.0*q_1*sin(q_2)^2 - 1.0*q_2*cos(q_2)) - 0.00052231*cos(q_3)*sin(q_4)*(1.0*q_1*sin(q_2)^2 - 1.0*q_2*cos(q_2))) - 0.4*cos(q_3)*(2.4552*sin(q_3)*(0.4*q_1*sin(q_2)^2 - 0.4*q_2*cos(q_2)) - 0.085735584*q_2*sin(q_2) - 0.065111904*sin(q_3)*(1.0*q_1*sin(q_2)^2 - 1.0*q_2*cos(q_2)) + cos(q_4)*(0.099708979*cos(q_4)*(1.0*q_2*sin(q_2) + 1.0*q_1*cos(q_2)*sin(q_2)) + 0.137576454*sin(q_3)*(1.0*q_1*sin(q_2)^2 - 1.0*q_2*cos(q_2)) + 0.099708979*cos(q_3)*sin(q_4)*(1.0*q_1*sin(q_2)^2 - 1.0*q_2*cos(q_2)) + 2.61155*cos(q_4)*sin(q_3)*(0.4*q_1*sin(q_2)^2 - 0.4*q_2*cos(q_2))) + 1.0*sin(q_4)*(0.099708979*sin(q_4)*(1.0*q_2*sin(q_2) + 1.0*q_1*cos(q_2)*sin(q_2)) - 0.00052231*sin(q_3)*(1.0*q_1*sin(q_2)^2 - 1.0*q_2*cos(q_2)) + 2.61155*sin(q_3)*sin(q_4)*(0.4*q_1*sin(q_2)^2 - 0.4*q_2*cos(q_2)) - 0.099708979*cos(q_3)*cos(q_4)*(1.0*q_1*sin(q_2)^2 - 1.0*q_2*cos(q_2))) - 0.085735584*q_1*cos(q_2)*sin(q_2)) - 1.0*cos(q_3)*(0.00636266901372*cos(q_4)*(1.0*q_2*sin(q_2) + 1.0*q_1*cos(q_2)*sin(q_2)) - 0.065111904*sin(q_3)*(0.4*q_1*sin(q_2)^2 - 0.4*q_2*cos(q_2)) + 0.0011000582042*sin(q_4)*(1.0*q_2*sin(q_2) + 1.0*q_1*cos(q_2)*sin(q_2)) + 0.00220370768768*q_2*sin(q_2) + 0.000142905064*cos(q_3)*(1.0*q_1*sin(q_2)^2 - 1.0*q_2*cos(q_2)) + 0.0610568292028*sin(q_3)*(1.0*q_1*sin(q_2)^2 - 1.0*q_2*cos(q_2)) - 0.00052231*sin(q_3)*sin(q_4)*(0.4*q_1*sin(q_2)^2 - 0.4*q_2*cos(q_2)) + 0.00220370768768*q_1*cos(q_2)*sin(q_2) - 0.0011000582042*cos(q_3)*cos(q_4)*(1.0*q_1*sin(q_2)^2 - 1.0*q_2*cos(q_2)) + 0.00636266901372*cos(q_3)*sin(q_4)*(1.0*q_1*sin(q_2)^2 - 1.0*q_2*cos(q_2)) + 0.137576454*cos(q_4)*sin(q_3)*(0.4*q_1*sin(q_2)^2 - 0.4*q_2*cos(q_2))) - 0.000122603128375*q_2*cos(q_2) - 0.002664500061125*q_2*sin(q_2) - sin(q_3)*(0.065111904*cos(q_3)*(0.4*q_1*sin(q_2)^2 - 0.4*q_2*cos(q_2)) + 1.0*cos(q_4)*(0.0009075152908*cos(q_4)*(1.0*q_2*sin(q_2) + 1.0*q_1*cos(q_2)*sin(q_2)) - 0.137576454*cos(q_3)*(0.4*q_1*sin(q_2)^2 - 0.4*q_2*cos(q_2)) + 0.04949441641494*sin(q_4)*(1.0*q_2*sin(q_2) + 1.0*q_1*cos(q_2)*sin(q_2)) - 0.0011399417958*sin(q_3)*(1.0*q_1*sin(q_2)^2 - 1.0*q_2*cos(q_2)) + 0.099708979*sin(q_3)*sin(q_4)*(0.4*q_1*sin(q_2)^2 - 0.4*q_2*cos(q_2)) - 0.04949441641494*cos(q_3)*cos(q_4)*(1.0*q_1*sin(q_2)^2 - 1.0*q_2*cos(q_2)) + 0.0009075152908*cos(q_3)*sin(q_4)*(1.0*q_1*sin(q_2)^2 - 1.0*q_2*cos(q_2))) - 1.0*sin(q_4)*(0.01524699328022*cos(q_4)*(1.0*q_2*sin(q_2) + 1.0*q_1*cos(q_2)*sin(q_2)) - 0.00052231*cos(q_3)*(0.4*q_1*sin(q_2)^2 - 0.4*q_2*cos(q_2)) - 0.0008524847092*sin(q_4)*(1.0*q_2*sin(q_2) + 1.0*q_1*cos(q_2)*sin(q_2)) + 0.00414266901372*sin(q_3)*(1.0*q_1*sin(q_2)^2 - 1.0*q_2*cos(q_2)) + 0.0008524847092*cos(q_3)*cos(q_4)*(1.0*q_1*sin(q_2)^2 - 1.0*q_2*cos(q_2)) + 0.01524699328022*cos(q_3)*sin(q_4)*(1.0*q_1*sin(q_2)^2 - 1.0*q_2*cos(q_2)) + 0.099708979*cos(q_4)*sin(q_3)*(0.4*q_1*sin(q_2)^2 - 0.4*q_2*cos(q_2))) + 0.000076501784*q_2*sin(q_2) - 0.00695065428736*cos(q_3)*(1.0*q_1*sin(q_2)^2 - 1.0*q_2*cos(q_2)) - 0.000242905064*sin(q_3)*(1.0*q_1*sin(q_2)^2 - 1.0*q_2*cos(q_2)) + 0.000076501784*q_1*cos(q_2)*sin(q_2)) - 0.002664500061125*q_1*cos(q_2)*sin(q_2);
c23=sin(q_3)*(0.000242905064*cos(q_3)*(q_2*sin(q_3) - 1.0*q_1*cos(q_3)*sin(q_2)) - 0.00695065428736*sin(q_3)*(q_2*sin(q_3) - 1.0*q_1*cos(q_3)*sin(q_2)) + 1.0*cos(q_4)*(0.0011399417958*cos(q_3)*(q_2*sin(q_3) - 1.0*q_1*cos(q_3)*sin(q_2)) + 0.0011399417958*sin(q_3)*(q_3 + q_1*cos(q_2)) - 0.04949441641494*cos(q_4)*(1.0*sin(q_3)*(q_2*sin(q_3) - 1.0*q_1*cos(q_3)*sin(q_2)) - 1.0*cos(q_3)*(q_3 + q_1*cos(q_2))) + 0.0009075152908*sin(q_4)*(1.0*sin(q_3)*(q_2*sin(q_3) - 1.0*q_1*cos(q_3)*sin(q_2)) - 1.0*cos(q_3)*(q_3 + q_1*cos(q_2)))) + 0.00695065428736*cos(q_3)*(q_3 + q_1*cos(q_2)) + 1.0*sin(q_4)*(0.00414266901372*cos(q_3)*(q_2*sin(q_3) - 1.0*q_1*cos(q_3)*sin(q_2)) + 0.00414266901372*sin(q_3)*(q_3 + q_1*cos(q_2)) - 0.0008524847092*cos(q_4)*(1.0*sin(q_3)*(q_2*sin(q_3) - 1.0*q_1*cos(q_3)*sin(q_2)) - 1.0*cos(q_3)*(q_3 + q_1*cos(q_2))) - 0.01524699328022*sin(q_4)*(1.0*sin(q_3)*(q_2*sin(q_3) - 1.0*q_1*cos(q_3)*sin(q_2)) - 1.0*cos(q_3)*(q_3 + q_1*cos(q_2)))) + 0.000242905064*sin(q_3)*(q_3 + q_1*cos(q_2))) - 1.0*cos(q_3)*(0.0610568292028*cos(q_3)*(q_2*sin(q_3) - 1.0*q_1*cos(q_3)*sin(q_2)) - 0.000142905064*sin(q_3)*(q_2*sin(q_3) - 1.0*q_1*cos(q_3)*sin(q_2)) + 0.000142905064*cos(q_3)*(q_3 + q_1*cos(q_2)) + 0.0610568292028*sin(q_3)*(q_3 + q_1*cos(q_2)) + 0.0011000582042*cos(q_4)*(1.0*sin(q_3)*(q_2*sin(q_3) - 1.0*q_1*cos(q_3)*sin(q_2)) - 1.0*cos(q_3)*(q_3 + q_1*cos(q_2))) - 0.00636266901372*sin(q_4)*(1.0*sin(q_3)*(q_2*sin(q_3) - 1.0*q_1*cos(q_3)*sin(q_2)) - 1.0*cos(q_3)*(q_3 + q_1*cos(q_2)))) + 0.4*sin(q_3)*(0.065111904*sin(q_3)*(q_2*sin(q_3) - 1.0*q_1*cos(q_3)*sin(q_2)) - 0.065111904*cos(q_3)*(q_3 + q_1*cos(q_2)) - 0.137576454*cos(q_4)*(1.0*sin(q_3)*(q_2*sin(q_3) - 1.0*q_1*cos(q_3)*sin(q_2)) - 1.0*cos(q_3)*(q_3 + q_1*cos(q_2))) + 0.00052231*sin(q_4)*(1.0*sin(q_3)*(q_2*sin(q_3) - 1.0*q_1*cos(q_3)*sin(q_2)) - 1.0*cos(q_3)*(q_3 + q_1*cos(q_2)))) + 0.4*cos(q_3)*(0.065111904*cos(q_3)*(q_2*sin(q_3) - 1.0*q_1*cos(q_3)*sin(q_2)) + 1.0*sin(q_4)*(0.00052231*cos(q_3)*(q_2*sin(q_3) - 1.0*q_1*cos(q_3)*sin(q_2)) + 0.00052231*sin(q_3)*(q_3 + q_1*cos(q_2)) - 0.099708979*cos(q_4)*(1.0*sin(q_3)*(q_2*sin(q_3) - 1.0*q_1*cos(q_3)*sin(q_2)) - 1.0*cos(q_3)*(q_3 + q_1*cos(q_2)))) - cos(q_4)*(0.137576454*cos(q_3)*(q_2*sin(q_3) - 1.0*q_1*cos(q_3)*sin(q_2)) + 0.137576454*sin(q_3)*(q_3 + q_1*cos(q_2)) - 0.099708979*sin(q_4)*(1.0*sin(q_3)*(q_2*sin(q_3) - 1.0*q_1*cos(q_3)*sin(q_2)) - 1.0*cos(q_3)*(q_3 + q_1*cos(q_2)))) + 0.065111904*sin(q_3)*(q_3 + q_1*cos(q_2)));
c24=- sin(q_3)*(1.0*sin(q_4)*(0.0008524847092*sin(q_4)*(cos(q_4)*(q_2*sin(q_3) - 1.0*q_1*cos(q_3)*sin(q_2)) + sin(q_4)*(q_3 + q_1*cos(q_2))) - 0.01524699328022*cos(q_4)*(cos(q_4)*(q_2*sin(q_3) - 1.0*q_1*cos(q_3)*sin(q_2)) + sin(q_4)*(q_3 + q_1*cos(q_2))) + 0.0008524847092*cos(q_4)*(q_2*cos(q_3) - 1.0*q_4 + q_1*sin(q_2)*sin(q_3)) + 0.01524699328022*sin(q_4)*(q_2*cos(q_3) - 1.0*q_4 + q_1*sin(q_2)*sin(q_3))) + 1.0*cos(q_4)*(0.0009075152908*cos(q_4)*(cos(q_4)*(q_2*sin(q_3) - 1.0*q_1*cos(q_3)*sin(q_2)) + sin(q_4)*(q_3 + q_1*cos(q_2))) + 0.04949441641494*sin(q_4)*(cos(q_4)*(q_2*sin(q_3) - 1.0*q_1*cos(q_3)*sin(q_2)) + sin(q_4)*(q_3 + q_1*cos(q_2))) + 0.04949441641494*cos(q_4)*(q_2*cos(q_3) - 1.0*q_4 + q_1*sin(q_2)*sin(q_3)) - 0.0009075152908*sin(q_4)*(q_2*cos(q_3) - 1.0*q_4 + q_1*sin(q_2)*sin(q_3)))) - 0.4*cos(q_3)*(cos(q_4)*(0.099708979*cos(q_4)*(cos(q_4)*(q_2*sin(q_3) - 1.0*q_1*cos(q_3)*sin(q_2)) + sin(q_4)*(q_3 + q_1*cos(q_2))) - 0.099708979*sin(q_4)*(q_2*cos(q_3) - 1.0*q_4 + q_1*sin(q_2)*sin(q_3))) + 1.0*sin(q_4)*(0.099708979*sin(q_4)*(cos(q_4)*(q_2*sin(q_3) - 1.0*q_1*cos(q_3)*sin(q_2)) + sin(q_4)*(q_3 + q_1*cos(q_2))) + 0.099708979*cos(q_4)*(q_2*cos(q_3) - 1.0*q_4 + q_1*sin(q_2)*sin(q_3)))) - 0.4*sin(q_3)*(0.00052231*cos(q_4)*(cos(q_4)*(q_2*sin(q_3) - 1.0*q_1*cos(q_3)*sin(q_2)) + sin(q_4)*(q_3 + q_1*cos(q_2))) + 0.137576454*sin(q_4)*(cos(q_4)*(q_2*sin(q_3) - 1.0*q_1*cos(q_3)*sin(q_2)) + sin(q_4)*(q_3 + q_1*cos(q_2))) + 0.137576454*cos(q_4)*(q_2*cos(q_3) - 1.0*q_4 + q_1*sin(q_2)*sin(q_3)) - 0.00052231*sin(q_4)*(q_2*cos(q_3) - 1.0*q_4 + q_1*sin(q_2)*sin(q_3))) - 1.0*cos(q_3)*(0.00636266901372*cos(q_4)*(cos(q_4)*(q_2*sin(q_3) - 1.0*q_1*cos(q_3)*sin(q_2)) + sin(q_4)*(q_3 + q_1*cos(q_2))) + 0.0011000582042*sin(q_4)*(cos(q_4)*(q_2*sin(q_3) - 1.0*q_1*cos(q_3)*sin(q_2)) + sin(q_4)*(q_3 + q_1*cos(q_2))) + 0.0011000582042*cos(q_4)*(q_2*cos(q_3) - 1.0*q_4 + q_1*sin(q_2)*sin(q_3)) - 0.00636266901372*sin(q_4)*(q_2*cos(q_3) - 1.0*q_4 + q_1*sin(q_2)*sin(q_3)));
c31=0;
c32=0.085735584*sin(q_3)*(0.4*q_1*sin(q_2)^2 - 0.4*q_2*cos(q_2)) - 0.0055242*cos(q_3)*(0.4*q_1*sin(q_2)^2 - 0.4*q_2*cos(q_2)) - 1.0*cos(q_4)*(0.01524699328022*cos(q_4)*(1.0*q_2*sin(q_2) + 1.0*q_1*cos(q_2)*sin(q_2)) - 0.00052231*cos(q_3)*(0.4*q_1*sin(q_2)^2 - 0.4*q_2*cos(q_2)) - 0.0008524847092*sin(q_4)*(1.0*q_2*sin(q_2) + 1.0*q_1*cos(q_2)*sin(q_2)) + 0.00414266901372*sin(q_3)*(1.0*q_1*sin(q_2)^2 - 1.0*q_2*cos(q_2)) + 0.0008524847092*cos(q_3)*cos(q_4)*(1.0*q_1*sin(q_2)^2 - 1.0*q_2*cos(q_2)) + 0.01524699328022*cos(q_3)*sin(q_4)*(1.0*q_1*sin(q_2)^2 - 1.0*q_2*cos(q_2)) + 0.099708979*cos(q_4)*sin(q_3)*(0.4*q_1*sin(q_2)^2 - 0.4*q_2*cos(q_2))) - sin(q_4)*(0.0009075152908*cos(q_4)*(1.0*q_2*sin(q_2) + 1.0*q_1*cos(q_2)*sin(q_2)) - 0.137576454*cos(q_3)*(0.4*q_1*sin(q_2)^2 - 0.4*q_2*cos(q_2)) + 0.04949441641494*sin(q_4)*(1.0*q_2*sin(q_2) + 1.0*q_1*cos(q_2)*sin(q_2)) - 0.0011399417958*sin(q_3)*(1.0*q_1*sin(q_2)^2 - 1.0*q_2*cos(q_2)) + 0.099708979*sin(q_3)*sin(q_4)*(0.4*q_1*sin(q_2)^2 - 0.4*q_2*cos(q_2)) - 0.04949441641494*cos(q_3)*cos(q_4)*(1.0*q_1*sin(q_2)^2 - 1.0*q_2*cos(q_2)) + 0.0009075152908*cos(q_3)*sin(q_4)*(1.0*q_1*sin(q_2)^2 - 1.0*q_2*cos(q_2))) - 0.00373631604328*q_2*sin(q_2) + 0.000216501784*cos(q_3)*(1.0*q_1*sin(q_2)^2 - 1.0*q_2*cos(q_2)) - 0.00234370768768*sin(q_3)*(1.0*q_1*sin(q_2)^2 - 1.0*q_2*cos(q_2)) - 0.00373631604328*q_1*cos(q_2)*sin(q_2);
c33=0.000216501784*cos(q_3)*(q_3 + q_1*cos(q_2)) - 0.000216501784*sin(q_3)*(q_2*sin(q_3) - 1.0*q_1*cos(q_3)*sin(q_2)) - 1.0*cos(q_4)*(0.00414266901372*cos(q_3)*(q_2*sin(q_3) - 1.0*q_1*cos(q_3)*sin(q_2)) + 0.00414266901372*sin(q_3)*(q_3 + q_1*cos(q_2)) - 0.0008524847092*cos(q_4)*(1.0*sin(q_3)*(q_2*sin(q_3) - 1.0*q_1*cos(q_3)*sin(q_2)) - 1.0*cos(q_3)*(q_3 + q_1*cos(q_2))) - 0.01524699328022*sin(q_4)*(1.0*sin(q_3)*(q_2*sin(q_3) - 1.0*q_1*cos(q_3)*sin(q_2)) - 1.0*cos(q_3)*(q_3 + q_1*cos(q_2)))) - 0.00234370768768*cos(q_3)*(q_2*sin(q_3) - 1.0*q_1*cos(q_3)*sin(q_2)) + sin(q_4)*(0.0011399417958*cos(q_3)*(q_2*sin(q_3) - 1.0*q_1*cos(q_3)*sin(q_2)) + 0.0011399417958*sin(q_3)*(q_3 + q_1*cos(q_2)) - 0.04949441641494*cos(q_4)*(1.0*sin(q_3)*(q_2*sin(q_3) - 1.0*q_1*cos(q_3)*sin(q_2)) - 1.0*cos(q_3)*(q_3 + q_1*cos(q_2))) + 0.0009075152908*sin(q_4)*(1.0*sin(q_3)*(q_2*sin(q_3) - 1.0*q_1*cos(q_3)*sin(q_2)) - 1.0*cos(q_3)*(q_3 + q_1*cos(q_2)))) - 0.00234370768768*sin(q_3)*(q_3 + q_1*cos(q_2));
c34=1.0*cos(q_4)*(0.0008524847092*sin(q_4)*(cos(q_4)*(q_2*sin(q_3) - 1.0*q_1*cos(q_3)*sin(q_2)) + sin(q_4)*(q_3 + q_1*cos(q_2))) - 0.01524699328022*cos(q_4)*(cos(q_4)*(q_2*sin(q_3) - 1.0*q_1*cos(q_3)*sin(q_2)) + sin(q_4)*(q_3 + q_1*cos(q_2))) + 0.0008524847092*cos(q_4)*(q_2*cos(q_3) - 1.0*q_4 + q_1*sin(q_2)*sin(q_3)) + 0.01524699328022*sin(q_4)*(q_2*cos(q_3) - 1.0*q_4 + q_1*sin(q_2)*sin(q_3))) - sin(q_4)*(0.0009075152908*cos(q_4)*(cos(q_4)*(q_2*sin(q_3) - 1.0*q_1*cos(q_3)*sin(q_2)) + sin(q_4)*(q_3 + q_1*cos(q_2))) + 0.04949441641494*sin(q_4)*(cos(q_4)*(q_2*sin(q_3) - 1.0*q_1*cos(q_3)*sin(q_2)) + sin(q_4)*(q_3 + q_1*cos(q_2))) + 0.04949441641494*cos(q_4)*(q_2*cos(q_3) - 1.0*q_4 + q_1*sin(q_2)*sin(q_3)) - 0.0009075152908*sin(q_4)*(q_2*cos(q_3) - 1.0*q_4 + q_1*sin(q_2)*sin(q_3)));
c41=0;
c42=0.00636266901372*cos(q_4)*(1.0*q_2*sin(q_2) + 1.0*q_1*cos(q_2)*sin(q_2)) + 0.0011000582042*sin(q_4)*(1.0*q_2*sin(q_2) + 1.0*q_1*cos(q_2)*sin(q_2)) + 0.05712763205872*sin(q_3)*(1.0*q_1*sin(q_2)^2 - 1.0*q_2*cos(q_2)) - 0.00052231*sin(q_3)*sin(q_4)*(0.4*q_1*sin(q_2)^2 - 0.4*q_2*cos(q_2)) - 0.0011000582042*cos(q_3)*cos(q_4)*(1.0*q_1*sin(q_2)^2 - 1.0*q_2*cos(q_2)) + 0.00636266901372*cos(q_3)*sin(q_4)*(1.0*q_1*sin(q_2)^2 - 1.0*q_2*cos(q_2)) + 0.137576454*cos(q_4)*sin(q_3)*(0.4*q_1*sin(q_2)^2 - 0.4*q_2*cos(q_2));
c43=0.05712763205872*cos(q_3)*(q_2*sin(q_3) - 1.0*q_1*cos(q_3)*sin(q_2)) + 0.05712763205872*sin(q_3)*(q_3 + q_1*cos(q_2)) + 0.0011000582042*cos(q_4)*(1.0*sin(q_3)*(q_2*sin(q_3) - 1.0*q_1*cos(q_3)*sin(q_2)) - 1.0*cos(q_3)*(q_3 + q_1*cos(q_2))) - 0.00636266901372*sin(q_4)*(1.0*sin(q_3)*(q_2*sin(q_3) - 1.0*q_1*cos(q_3)*sin(q_2)) - 1.0*cos(q_3)*(q_3 + q_1*cos(q_2)));
c44=0.00636266901372*cos(q_4)*(cos(q_4)*(q_2*sin(q_3) - 1.0*q_1*cos(q_3)*sin(q_2)) + sin(q_4)*(q_3 + q_1*cos(q_2))) + 0.0011000582042*sin(q_4)*(cos(q_4)*(q_2*sin(q_3) - 1.0*q_1*cos(q_3)*sin(q_2)) + sin(q_4)*(q_3 + q_1*cos(q_2))) + 0.0011000582042*cos(q_4)*(q_2*cos(q_3) - 1.0*q_4 + q_1*sin(q_2)*sin(q_3)) - 0.00636266901372*sin(q_4)*(q_2*cos(q_3) - 1.0*q_4 + q_1*sin(q_2)*sin(q_3));

C=[c11 c12 c13 c14;c21 c22 c23 c24;c31 c32 c33 c34;c41 c42 c43 c44];

Kp = 30;
Kd = 10;

acc = q_des_ddot - Kp*(q - q_des) - Kd*(q_dot - q_des_dot)
torque = M*acc + C*q_dot;
